simulink model "sedemo_shared_buffer_mgmt"  (Simulink 7.5)
settings: Solver=VariableStepDiscrete  StartTime=0.0  StopTime=10  MaxStep=inf  RelTol=1e-3
undefined symbols (not defined in the file or in its folder): des_subsystemblock, des_subsysteminport, des_subsystemoutport, des_subsystemsupportblock
libraries: simeventstranslate1 x25, simeventssink1 x23, simeventsrouting1 x9, simeventsgates1 x6, simeventsattributes2 x6, simeventsgenerators1 x6, simeventsserver1 x3, simeventsqueue1 x2, simulink x1, simeventsinfo x1
(part 1 of 4)
settings Model: Creator=The MathWorks Inc.  ExtModeAutoUpdateStatusClock=off
settings DataIOCC: SaveOutput=off  SignalLogging=off  SaveTime=off
settings OptimizationCC: InitFltsAndDblsToZero=on
settings DebuggingCC: AlgebraicLoopMsg=error  SolverPrmCheckMsg=none  StrictBusMsg=Warning
settings GRTTargetCC: TargetFcnLib=ansi_tfl_tmw_new.mat
settings SimEventsCC: propDiagAttribOutput=0  propDiagFcnCallOutput=1  propDiagStatOutput=0

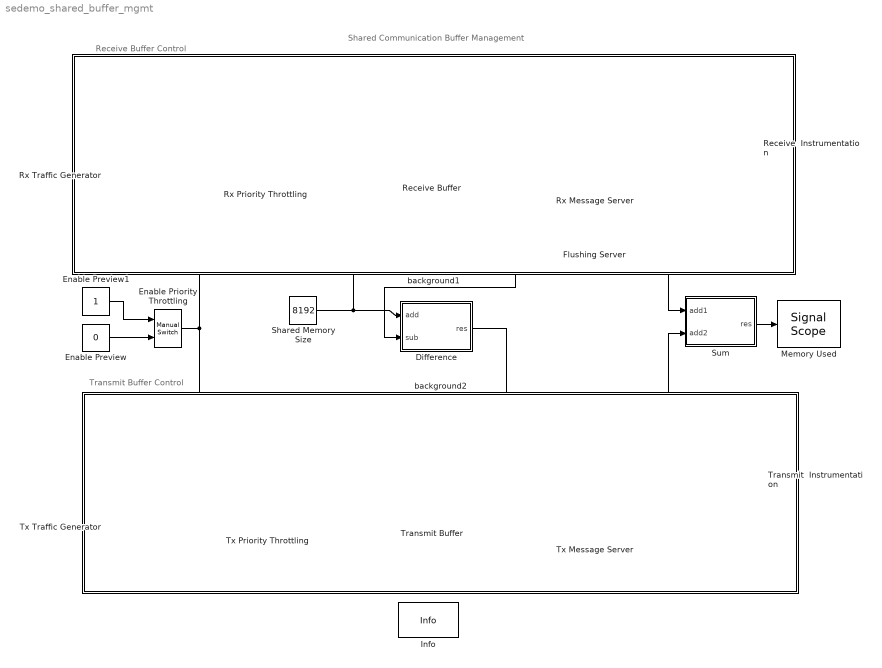
== system sedemo_shared_buffer_mgmt ==
  note: Shared Communication Buffer Management
  note: Receive Buffer Control
  note: Transmit Buffer Control
  Difference : Subsystem  LoadFcn=des_subsystemblock(gcb, 'load');  InitFcn=des_subsystemblock(gcb, 'init');  StartFcn=des_subsystemblock(gcb, 'start');  StopFcn=des_subsystemblock(gcb, 'stop');
      settings: CopyFcn=des_subsystemblock(gcb, 'copy');  DeleteFcn=des_subsystemblock(gcb, 'delete');  UndoDeleteFcn=des_subsystemblock(gcb, 'undodelete');  ModelCloseFcn=des_subsystemblock(gcb, 'modelclose');  PreSaveFcn=des_subsystemblock(gcb, 'presave');  NameChangeFcn=des_subsystemblock(gcb, 'namechange');  ParentCloseFcn=des_subsystemblock(gcb, 'parentclose');  ErrorFcn=des_subsystemerror
  Enable Preview : Constant  Value=0  OutDataType=sfix(16)  OutScaling=2^0
  Enable Preview1 : Constant  OutDataType=sfix(16)  OutScaling=2^0
  Enable Priority Throttling : simulink/Signal Routing/Manual Switch  SystemSampleTime=-1  sw=1  action=0  varsize=off
  Flushing Server : simeventsserver1/Single Server  Priority=1  SystemSampleTime=-1  ServiceTimeFrom=Dialog  ServiceTime=.01  AttributeName=ServiceTime  PriorityServiceCompletion=500  PermitPreemption=off  SortingAttributeName=PriorityAttributeName  SortingDirection=Ascending  WriteToAttribute=off  ResidualAttributeName=ResidualServiceTime  CreateAttribute=on  EnableTOPort=off  StatNumberDeparted=Off  StatNumberInBlock=Off  StatNumberPreempted=Off  StatPendingEntity=Off  StatAverageWait=Off  StatUtilization=Off  StatNumberTimedout=Off
  Info : simeventsinfo/Info  SystemSampleTime=-1
  Memory Used : simeventssink1/Signal Scope  Priority=1  SystemSampleTime=-1  PlotType=Stair  InputType=Signal  NumInputs=1  AttributeNameY=Count  XInputOptionSignal=Event time  XInputOptionEntity=Event time  AttributeNameX=Count  EnableEntityOutport=on  XMin=-0.1  XMax=10.1  XLimitExceededOption=Stretch axis limits  YLimitExceededOption=Stretch axis limits  AxisGrid=on  AxisLegend=off  LineDisables=""  LineColors="1  0  0"  LineStyles=-  LineMarkers=None  OpenScopeAtSimStart=on  Title=Total Memory Used  YLabel=Memory  XLabel=Time  FigurePosition=[598 478 273 129]  AxisZoom=off  DataStoreOption=Limited  DataPointsLimit=10000  StatNumberArrived=Off  ShowCountPlotted=off  ShowToolbar=off
      settings: YMin=-1.09  YMax=10
  Receive  Instrumentation : Subsystem
  Receive Buffer : Subsystem  mask(Variable Capacity, Variable Space per Entity Buffer){attribNameLength=space, thresholdLow=.35, thresholdHigh=.55}
      mask prompts: attribNameLength "Entity space from attribute:"; thresholdLow "Low threshold (fraction):"; thresholdHigh "High threshold (fraction):"
      mask help: Variable capacity queue that allows entities to occupy a variable amount of space per entitiy. The amount of space from an entity is specified from the attribute named in the dialog.
      mask init:
      | % Get attribute name to use for space needed for each entity
      | % and use it to set the attribute name for 'Get Attribute'
      | % and 'Get Attribute1' block
      | name = get_param(gcb,'attribNameLength');
      | set_param([gcb '/Get Attribute'],'AttributeName',name);
      | set_param([gcb '/Get Attribute1'],'AttributeName',name);
      mask Display:
      | color('blue')
      | text(35,67,'Variable Space\nper Entity and\nFlushing')
  Rx Message Server : simeventsserver1/Single Server  Priority=1  SystemSampleTime=-1  ServiceTimeFrom=Dialog  ServiceTime=.23  AttributeName=ServiceTime  PriorityServiceCompletion=500  PermitPreemption=off  SortingAttributeName=PriorityAttributeName  SortingDirection=Ascending  WriteToAttribute=off  ResidualAttributeName=ResidualServiceTime  CreateAttribute=on  EnableTOPort=off  StatNumberDeparted=On  StatNumberInBlock=Off  StatNumberPreempted=Off  StatPendingEntity=Off  StatAverageWait=Off  StatUtilization=Off  StatNumberTimedout=Off
  Rx Priority Throttling : Subsystem
  Rx Traffic Generator : Subsystem
  Shared Memory Size : Constant  Value=8192  OutDataType=sfix(16)  OutScaling=2^0
  Sum : Subsystem  LoadFcn=des_subsystemblock(gcb, 'load');  InitFcn=des_subsystemblock(gcb, 'init');  StartFcn=des_subsystemblock(gcb, 'start');  StopFcn=des_subsystemblock(gcb, 'stop');
      settings: CopyFcn=des_subsystemblock(gcb, 'copy');  DeleteFcn=des_subsystemblock(gcb, 'delete');  UndoDeleteFcn=des_subsystemblock(gcb, 'undodelete');  ModelCloseFcn=des_subsystemblock(gcb, 'modelclose');  PreSaveFcn=des_subsystemblock(gcb, 'presave');  NameChangeFcn=des_subsystemblock(gcb, 'namechange');  ParentCloseFcn=des_subsystemblock(gcb, 'parentclose');  ErrorFcn=des_subsystemerror
  Transmit  Instrumentation : Subsystem
  Transmit Buffer : Subsystem  mask(Variable Capacity, Variable Space per Entity Buffer){attribNameLength=space, thresholdLow=.4, thresholdHigh=.6}
      mask prompts: attribNameLength "Entity space from attribute:"; thresholdLow "Low threshold (fraction):"; thresholdHigh "High threshold (fraction):"
      mask help: Variable capacity queue that allows entities to occupy a variable amount of space per entitiy. The amount of space from an entity is specified from the attribute named in the dialog.
      mask init: same as sedemo_shared_buffer_mgmt/Receive Buffer
      mask Display:
      | color('blue')
      | text(35,67,'Variable Capacity\nwith Variable Space\nper Entity')
  Tx Message Server : simeventsserver1/Single Server  Priority=1  SystemSampleTime=-1  ServiceTimeFrom=Dialog  ServiceTime=.23  AttributeName=ServiceTime  PriorityServiceCompletion=500  PermitPreemption=off  SortingAttributeName=PriorityAttributeName  SortingDirection=Ascending  WriteToAttribute=off  ResidualAttributeName=ResidualServiceTime  CreateAttribute=on  EnableTOPort=off  StatNumberDeparted=On  StatNumberInBlock=Off  StatNumberPreempted=Off  StatPendingEntity=Off  StatAverageWait=Off  StatUtilization=Off  StatNumberTimedout=Off
  Tx Priority Throttling : Subsystem
  Tx Traffic Generator : Subsystem
  background1 : Subsystem
      mask Display: disp('')
  background2 : Subsystem
      mask Display: disp('')
  wires:
  Rx Message Server/1 -> Receive  Instrumentation/6(Num Served)
  Receive Buffer/1(#n) -> Receive  Instrumentation/1(Msgs)
  Receive Buffer/2(Mem) -> Receive  Instrumentation/2(Mem Used), Sum/1(add1), Difference/2(sub)
  Receive Buffer/3(high) -> Receive  Instrumentation/3(High), Rx Priority Throttling/3(drop high)
  Receive Buffer/4(#fl) -> Receive  Instrumentation/4(Num fl)
  Receive Buffer/5(low) -> Rx Priority Throttling/1(drop low), Receive  Instrumentation/5(low)
  Tx Message Server/1 -> Transmit  Instrumentation/6(Num Served)
  Transmit Buffer/1(#n) -> Transmit  Instrumentation/1(Msgs)
  Transmit Buffer/2(Mem) -> Sum/2(add2), Transmit  Instrumentation/2(Mem Used)
  Transmit Buffer/3(high) -> Tx Priority Throttling/3(drop high), Transmit  Instrumentation/3(high)
  Transmit Buffer/4(#fl) -> Transmit  Instrumentation/4(Num fl)
  Transmit Buffer/5(low) -> Tx Priority Throttling/1(drop low), Transmit  Instrumentation/5(low)
  Difference/1(res) -> Transmit Buffer/1(cap), Transmit  Instrumentation/7(Thresh)
  Sum/1(res) -> Memory Used/1
  Shared Memory Size/1 -> Difference/1(add), Receive Buffer/1(cap), Receive  Instrumentation/7(Thresh)
  Enable Preview1/1 -> Enable Priority Throttling/1
  Enable Preview/1 -> Enable Priority Throttling/2
  Enable Priority Throttling/1 -> Rx Priority Throttling/2(enable), Tx Priority Throttling/2(enable)
  connections:
  Receive Buffer/RConn1 -- Rx Message Server/LConn1
  Receive  Instrumentation/LConn1 -- Rx Message Server/RConn1
  Rx Traffic Generator/RConn1 -- Rx Priority Throttling/LConn1
  Rx Priority Throttling/RConn1 -- Receive Buffer/LConn1
  Transmit  Instrumentation/LConn1 -- Tx Message Server/RConn1
  Transmit Buffer/RConn1 -- Tx Message Server/LConn1
  Tx Traffic Generator/RConn1 -- Tx Priority Throttling/LConn1
  Tx Priority Throttling/RConn1 -- Transmit Buffer/LConn1
  Receive Buffer/RConn2 -- Flushing Server/LConn1
  Flushing Server/RConn1 -- Receive  Instrumentation/LConn2

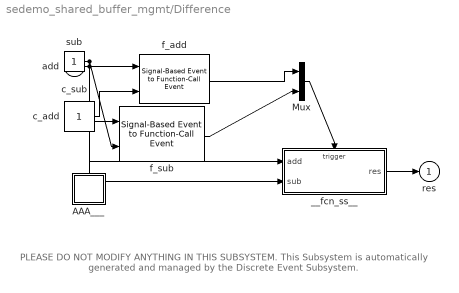
== system sedemo_shared_buffer_mgmt/Difference ==
  note: PLEASE DO NOT MODIFY ANYTHING IN THIS SUBSYSTEM.
      | This Subsystem is automatically generated and
      | managed by the Discrete Event Subsystem.
  add : Inport  DataType=double  OutDataType=sfix(16)  OutScaling=2^0  OutDataTypeStr=double
  sub : Inport  Port=2  DataType=double  OutDataType=sfix(16)  OutScaling=2^0  OutDataTypeStr=double
  AAA___ : Subsystem  LoadFcn=des_subsystemsupportblock(gcb, 'load');  InitFcn=des_subsystemsupportblock(gcb, 'init');  StartFcn=des_subsystemsupportblock(gcb, 'start');  StopFcn=des_subsystemsupportblock(gcb, 'stop');
      settings: CopyFcn=des_subsystemsupportblock(gcb, 'copy');  DeleteFcn=des_subsystemsupportblock(gcb, 'delete');  UndoDeleteFcn=des_subsystemsupportblock(gcb, 'undodelete');  ModelCloseFcn=des_subsystemsupportblock(gcb, 'modelclose');  PreSaveFcn=des_subsystemsupportblock(gcb, 'presave');  NameChangeFcn=des_subsystemsupportblock(gcb, 'namechange');  OpenFcn=des_subsystemsupportblock(gcb, 'open');  ParentCloseFcn=des_subsystemsupportblock(gcb, 'parentclose');
  Mux : Mux  Inputs=2
  __fcn_ss__ : Subsystem  TreatAsAtomicUnit=on
      settings: PropExecContextOutsideSubsystem=on
  c_add : Constant  OutDataType=sfix(16)  OutScaling=2^0
  c_sub : Constant  OutDataType=sfix(16)  OutScaling=2^0
  f_add : simeventstranslate1/Signal-Based Event to Function-Call Event  Priority=1  SystemSampleTime=-1  GenerateFunctionCallUpon=Sample time hit from port ts  SignalEdgeOption=Rising  EnableE1Port=on  EnableF2Port=off  EnableE2Port=off  SpecifyEventPriority=off  PriorityFunctionCall=20  FunctionCallDelayFrom=Dialog  DelayFunctionCall=0  StatNumberF1Calls=Off  StatNumberF2Calls=Off  MaskBlockType=DESS_EVENT_PORT
  f_sub : simeventstranslate1/Signal-Based Event to Function-Call Event  Priority=1  SystemSampleTime=-1  GenerateFunctionCallUpon=Sample time hit from port ts  SignalEdgeOption=Rising  EnableE1Port=on  EnableF2Port=off  EnableE2Port=off  SpecifyEventPriority=off  PriorityFunctionCall=20  FunctionCallDelayFrom=Dialog  DelayFunctionCall=0  StatNumberF1Calls=Off  StatNumberF2Calls=Off  MaskBlockType=DESS_EVENT_PORT
  res : Outport  OutDataType=sfix(16)  OutScaling=2^0
  wires:
  __fcn_ss__/1(res) -> res/1
  f_add/1 -> Mux/1
  c_add/1 -> f_add/2
  Mux/1 -> __fcn_ss__/Trigger
  f_sub/1 -> Mux/2
  c_sub/1 -> f_sub/2
  add/1 -> f_add/1, __fcn_ss__/1(add)
  sub/1 -> f_sub/1, __fcn_ss__/2(sub)

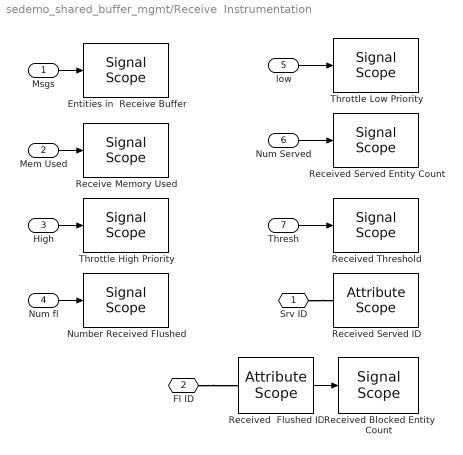
== system sedemo_shared_buffer_mgmt/Receive  Instrumentation ==
  Msgs : Inport  OutDataType=sfix(16)  OutScaling=2^0
  Mem Used : Inport  Port=2  OutDataType=sfix(16)  OutScaling=2^0
  High : Inport  Port=3  OutDataType=sfix(16)  OutScaling=2^0
  Num fl : Inport  Port=4  OutDataType=sfix(16)  OutScaling=2^0
  low : Inport  Port=5  OutDataType=sfix(16)  OutScaling=2^0
  Num Served : Inport  Port=6  OutDataType=sfix(16)  OutScaling=2^0
  Thresh : Inport  Port=7  OutDataType=sfix(16)  OutScaling=2^0
  Entities in  Receive Buffer : simeventssink1/Signal Scope  Priority=1  SystemSampleTime=-1  PlotType=Stair  InputType=Signal  NumInputs=1  AttributeNameY=Count  XInputOptionSignal=Event time  XInputOptionEntity=Event time  AttributeNameX=Count  EnableEntityOutport=on  XMin=0  XMax=10  XLimitExceededOption=Stretch axis limits  YLimitExceededOption=Stretch axis limits  AxisGrid=on  AxisLegend=off  LineDisables=""  LineColors=b  LineStyles=-  LineMarkers=.  OpenScopeAtSimStart=on  Title=Messages in Receive Buffer  YLabel=Num. Messages  XLabel=Time  FigurePosition=[28 477 268 129]  AxisZoom=off  DataStoreOption=Limited  DataPointsLimit=10000  StatNumberArrived=Off  ShowCountPlotted=off  ShowToolbar=off
      settings: YMin=0  YMax=10
  Number Received Flushed : simeventssink1/Signal Scope  Priority=1  SystemSampleTime=-1  PlotType=Stair  InputType=Signal  NumInputs=1  AttributeNameY=Count  XInputOptionSignal=Event time  XInputOptionEntity=Event time  AttributeNameX=Count  EnableEntityOutport=on  XMin=0  XMax=10  XLimitExceededOption=Stretch axis limits  YLimitExceededOption=Stretch axis limits  AxisGrid=on  AxisLegend=off  LineDisables=""  LineColors="1  0  0"  LineStyles=-  LineMarkers=None  OpenScopeAtSimStart=off  Title=Number Received Entities Flushed  YLabel=Number Flushed  XLabel=Time  FigurePosition=[883 418 268 129]  AxisZoom=off  DataStoreOption=Limited  DataPointsLimit=10000  StatNumberArrived=Off  ShowCountPlotted=off  ShowToolbar=on
      settings: YMin=0  YMax=10
  Receive Memory Used : simeventssink1/Signal Scope  Priority=1  SystemSampleTime=-1  PlotType=Stair  InputType=Signal  NumInputs=1  AttributeNameY=Count  XInputOptionSignal=Event time  XInputOptionEntity=Event time  AttributeNameX=Count  EnableEntityOutport=on  XMin=-0.1  XMax=10.1  XLimitExceededOption=Stretch axis limits  YLimitExceededOption=Stretch axis limits  AxisGrid=on  AxisLegend=off  LineDisables=""  LineColors="1  0  0"  LineStyles=-  LineMarkers=None  OpenScopeAtSimStart=on  Title=Receive Memory Used  YLabel=Memory  XLabel=Time  FigurePosition=[304 478 285 129]  AxisZoom=off  DataStoreOption=Limited  DataPointsLimit=10000  StatNumberArrived=Off  ShowCountPlotted=off  ShowToolbar=off
      settings: YMin=-1.09  YMax=10
  Received  Flushed ID : simeventssink1/Attribute Scope  Priority=1  SystemSampleTime=-1  PlotType=Stair  InputType=Attribute  NumInputs=1  AttributeNameY=count  XInputOptionSignal=Event time  XInputOptionEntity=Event time  AttributeNameX=Count  EnableEntityOutport=off  XMin=0  XMax=10  XLimitExceededOption=Stretch axis limits  YLimitExceededOption=Stretch axis limits  AxisGrid=on  AxisLegend=off  LineDisables=""  LineColors=b  LineStyles=-  LineMarkers=.  OpenScopeAtSimStart=off  Title=ID of Received Entities Flushed  YLabel=ID  XLabel=Time  FigurePosition=[783 206 237 129]  AxisZoom=off  DataStoreOption=Limited  DataPointsLimit=10000  StatNumberArrived=On  ShowCountPlotted=off  ShowToolbar=on
      settings: YMin=0  YMax=10
  Received Blocked Entity Count : simeventssink1/Signal Scope  Priority=1  SystemSampleTime=-1  PlotType=Stair  InputType=Signal  NumInputs=1  AttributeNameY=Count  XInputOptionSignal=Event time  XInputOptionEntity=Event time  AttributeNameX=Count  EnableEntityOutport=on  XMin=-0.1  XMax=10.1  XLimitExceededOption=Stretch axis limits  YLimitExceededOption=Stretch axis limits  AxisGrid=on  AxisLegend=off  LineDisables=""  LineColors=b  LineStyles=-  LineMarkers=.  OpenScopeAtSimStart=off  Title=Received Flushed Entity Count  YLabel=Entities Flushed  XLabel=Time  FigurePosition=[596 206 280 129]  AxisZoom=off  DataStoreOption=Limited  DataPointsLimit=10000  StatNumberArrived=Off  ShowCountPlotted=off  ShowToolbar=on
      settings: YMin=-0.19  YMax=19.19
  Received Served Entity Count : simeventssink1/Signal Scope  Priority=1  SystemSampleTime=-1  PlotType=Stair  InputType=Signal  NumInputs=1  AttributeNameY=Count  XInputOptionSignal=Event time  XInputOptionEntity=Event time  AttributeNameX=Count  EnableEntityOutport=on  XMin=0  XMax=10  XLimitExceededOption=Stretch axis limits  YLimitExceededOption=Stretch axis limits  AxisGrid=on  AxisLegend=off  LineDisables=""  LineColors=b  LineStyles=-  LineMarkers=.  OpenScopeAtSimStart=off  Title=Received Served Entity Count  YLabel=Entities Served  XLabel=Time  FigurePosition=[596 418 279 129]  AxisZoom=off  DataStoreOption=Limited  DataPointsLimit=10000  StatNumberArrived=Off  ShowCountPlotted=off  ShowToolbar=on
      settings: YMin=0  YMax=10
  Received Served ID : simeventssink1/Attribute Scope  Priority=1  SystemSampleTime=-1  PlotType=Stair  InputType=Attribute  NumInputs=1  AttributeNameY=count  XInputOptionSignal=Event time  XInputOptionEntity=Event time  AttributeNameX=Count  EnableEntityOutport=off  XMin=0  XMax=10  XLimitExceededOption=Stretch axis limits  YLimitExceededOption=Stretch axis limits  AxisGrid=on  AxisLegend=off  LineDisables=""  LineColors=b  LineStyles=-  LineMarkers=.  OpenScopeAtSimStart=off  Title=ID of Receive Entities Served  YLabel=ID  XLabel=Time  FigurePosition=[884 206 243 129]  AxisZoom=off  DataStoreOption=Limited  DataPointsLimit=10000  StatNumberArrived=Off  ShowCountPlotted=off  ShowToolbar=on
      settings: YMin=0  YMax=10
  Received Threshold : simeventssink1/Signal Scope  Priority=1  SystemSampleTime=-1  PlotType=Stair  InputType=Signal  NumInputs=1  AttributeNameY=Count  XInputOptionSignal=Event time  XInputOptionEntity=Event time  AttributeNameX=Count  EnableEntityOutport=on  XMin=0  XMax=10  XLimitExceededOption=Stretch axis limits  YLimitExceededOption=Stretch axis limits  AxisGrid=on  AxisLegend=off  LineDisables=""  LineColors="1  0  0"  LineStyles=-  LineMarkers=None  OpenScopeAtSimStart=off  Title=Threshold for Transmit Memory Used  YLabel=Threshold  XLabel=Time  FigurePosition=[27 206 272 129]  AxisZoom=off  DataStoreOption=Limited  DataPointsLimit=10000  StatNumberArrived=Off  ShowCountPlotted=off  ShowToolbar=on
      settings: YMin=0  YMax=10
  Throttle High Priority : simeventssink1/Signal Scope  Priority=1  SystemSampleTime=-1  PlotType=Stair  InputType=Signal  NumInputs=1  AttributeNameY=Count  XInputOptionSignal=Event time  XInputOptionEntity=Event time  AttributeNameX=Count  EnableEntityOutport=on  XMin=0  XMax=10  XLimitExceededOption=Stretch axis limits  YLimitExceededOption=Stretch axis limits  AxisGrid=on  AxisLegend=off  LineDisables=""  LineColors="1  0  0"  LineStyles=-  LineMarkers=None  OpenScopeAtSimStart=off  Title=Throttle High Priority Messages  YLabel=Enable Flush  XLabel=Time  FigurePosition=[303 418 283 129]  AxisZoom=off  DataStoreOption=Limited  DataPointsLimit=10000  StatNumberArrived=Off  ShowCountPlotted=off  ShowToolbar=on
      settings: YMin=0  YMax=10
  Throttle Low Priority : simeventssink1/Signal Scope  Priority=1  SystemSampleTime=-1  PlotType=Stair  InputType=Signal  NumInputs=1  AttributeNameY=Count  XInputOptionSignal=Event time  XInputOptionEntity=Event time  AttributeNameX=Count  EnableEntityOutport=on  XMin=0  XMax=10  XLimitExceededOption=Stretch axis limits  YLimitExceededOption=Stretch axis limits  AxisGrid=on  AxisLegend=off  LineDisables=""  LineColors="1  0  0"  LineStyles=-  LineMarkers=None  OpenScopeAtSimStart=off  Title=Throttle Low Priority Message  YLabel=Status  XLabel=Time  FigurePosition=[307 418 268 129]  AxisZoom=off  DataStoreOption=Limited  DataPointsLimit=10000  StatNumberArrived=Off  ShowCountPlotted=off  ShowToolbar=on
      settings: YMin=0  YMax=10
  Srv ID : PMIOPort  Port=1  Side=Left
  Fl ID : PMIOPort  Port=2  Side=Left
  wires:
  Received  Flushed ID/1 -> Received Blocked Entity Count/1
  low/1 -> Throttle Low Priority/1
  Thresh/1 -> Received Threshold/1
  Mem Used/1 -> Receive Memory Used/1
  Msgs/1 -> Entities in  Receive Buffer/1
  High/1 -> Throttle High Priority/1
  Num fl/1 -> Number Received Flushed/1
  Num Served/1 -> Received Served Entity Count/1
  connections:
  Srv ID/RConn1 -- Received Served ID/LConn1
  Fl ID/RConn1 -- Received  Flushed ID/LConn1

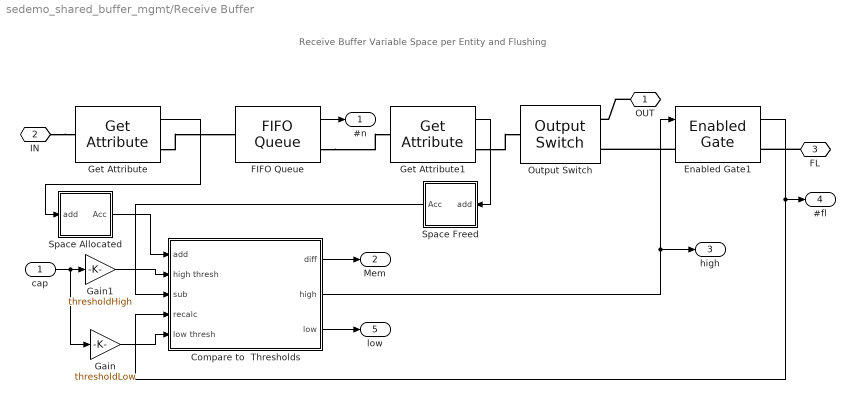
== system sedemo_shared_buffer_mgmt/Receive Buffer ==
  note: Receive Buffer
      | Variable Space per Entity and Flushing
  cap : Inport  OutDataType=sfix(16)  OutScaling=2^0
  Compare to  Thresholds : Subsystem  LoadFcn=des_subsystemblock(gcb, 'load');  InitFcn=des_subsystemblock(gcb, 'init');  StartFcn=des_subsystemblock(gcb, 'start');  StopFcn=des_subsystemblock(gcb, 'stop');
      settings: CopyFcn=des_subsystemblock(gcb, 'copy');  DeleteFcn=des_subsystemblock(gcb, 'delete');  UndoDeleteFcn=des_subsystemblock(gcb, 'undodelete');  ModelCloseFcn=des_subsystemblock(gcb, 'modelclose');  PreSaveFcn=des_subsystemblock(gcb, 'presave');  NameChangeFcn=des_subsystemblock(gcb, 'namechange');  ParentCloseFcn=des_subsystemblock(gcb, 'parentclose');  ErrorFcn=des_subsystemerror
  Enabled Gate1 : simeventsgates1/Enabled Gate  Priority=1  SystemSampleTime=-1  SpecifyEventPriority=off  PriorityGateEnableOpenClose=500  StatNumberDeparted=On
  FIFO Queue : simeventsqueue1/FIFO Queue  Priority=1  SystemSampleTime=-1  Capacity=inf  EnableTOPort=off  StatNumberDeparted=Off  StatNumberInBlock=On  StatPendingEntity=Off  StatAverageWait=Off  StatAverageQueueLength=Off  StatNumberTimedout=Off
  Gain : Gain  Gain=thresholdLow  ParameterDataType=sfix(16)  ParameterScaling=2^0  OutDataType=sfix(16)  OutScaling=2^0
  Gain1 : Gain  Gain=thresholdHigh  ParameterDataType=sfix(16)  ParameterScaling=2^0  OutDataType=sfix(16)  OutScaling=2^0
  Get Attribute : simeventsattributes2/Get Attribute  Priority=1  DialogController=des_ddg_create  DialogControllerArgs=DataTag41  SystemSampleTime=-1  AttributeName=space  AttributeMissing=Error  AttributeDefaultValue=1  AttributeSendTiming=After entity departure  AttributeTreatAsVector=1  StatNumberDeparted=Off  EvaluatedDefaultAttributeValue={[]}
  Get Attribute1 : simeventsattributes2/Get Attribute  Priority=1  DialogController=des_ddg_create  DialogControllerArgs=DataTag43  SystemSampleTime=-1  AttributeName=space  AttributeMissing=Error  AttributeDefaultValue=1  AttributeSendTiming=After entity departure  AttributeTreatAsVector=1  StatNumberDeparted=Off  EvaluatedDefaultAttributeValue={[]}
  Output Switch : simeventsrouting1/Output Switch  Priority=1  SystemSampleTime=-1  NumberOutputPorts=2  SwitchingCriterion=First port that is not blocked  InitialSeed=34567  AttributeName=Attribute1  InitialConditionsOpt=on  InitialConditions=1  EntityBufferOpt=on  SpecifyEventPriority=off  PriorityOutputSwitchSelectPort=4100  TimeoutPortOpt=off  StatNumberDeparted=Off  StatNumberTimedOut=Off  StatPendingEntity=Off  StatLastDeparturePort=Off  EvaluatedNumPorts=2
  Space Allocated : Subsystem  LoadFcn=des_subsystemblock(gcb, 'load');  InitFcn=des_subsystemblock(gcb, 'init');  StartFcn=des_subsystemblock(gcb, 'start');  StopFcn=des_subsystemblock(gcb, 'stop');
      settings: CopyFcn=des_subsystemblock(gcb, 'copy');  DeleteFcn=des_subsystemblock(gcb, 'delete');  UndoDeleteFcn=des_subsystemblock(gcb, 'undodelete');  ModelCloseFcn=des_subsystemblock(gcb, 'modelclose');  PreSaveFcn=des_subsystemblock(gcb, 'presave');  NameChangeFcn=des_subsystemblock(gcb, 'namechange');  ParentCloseFcn=des_subsystemblock(gcb, 'parentclose');  ErrorFcn=des_subsystemerror
  Space Freed : Subsystem  LoadFcn=des_subsystemblock(gcb, 'load');  InitFcn=des_subsystemblock(gcb, 'init');  StartFcn=des_subsystemblock(gcb, 'start');  StopFcn=des_subsystemblock(gcb, 'stop');
      settings: CopyFcn=des_subsystemblock(gcb, 'copy');  DeleteFcn=des_subsystemblock(gcb, 'delete');  UndoDeleteFcn=des_subsystemblock(gcb, 'undodelete');  ModelCloseFcn=des_subsystemblock(gcb, 'modelclose');  PreSaveFcn=des_subsystemblock(gcb, 'presave');  NameChangeFcn=des_subsystemblock(gcb, 'namechange');  ParentCloseFcn=des_subsystemblock(gcb, 'parentclose');  ErrorFcn=des_subsystemerror
  OUT : PMIOPort  Port=1  Side=Right
  IN : PMIOPort  Port=2  Side=Left
  FL : PMIOPort  Port=3  Side=Right
  #n : Outport  OutDataType=sfix(16)  OutScaling=2^0
  Mem : Outport  Port=2  OutDataType=sfix(16)  OutScaling=2^0
  high : Outport  Port=3  OutDataType=sfix(16)  OutScaling=2^0
  #fl : Outport  Port=4  OutDataType=sfix(16)  OutScaling=2^0
  low : Outport  Port=5  OutDataType=sfix(16)  OutScaling=2^0
  wires:
  Get Attribute1/1 -> Space Freed/1(add)
  Get Attribute/1 -> Space Allocated/1(add)
  Space Freed/1(Acc) -> Compare to  Thresholds/3(sub)
  Space Allocated/1(Acc) -> Compare to  Thresholds/1(add)
  Compare to  Thresholds/2(high) -> Enabled Gate1/1, high/1
  Enabled Gate1/1 -> Compare to  Thresholds/4(recalc), #fl/1
  FIFO Queue/1 -> #n/1
  Compare to  Thresholds/1(diff) -> Mem/1
  Gain/1 -> Compare to  Thresholds/5(low thresh)
  Compare to  Thresholds/3(low) -> low/1
  cap/1 -> Gain/1, Gain1/1
  Gain1/1 -> Compare to  Thresholds/2(high thresh)
  connections:
  Enabled Gate1/LConn1 -- Output Switch/RConn2
  Get Attribute/RConn1 -- FIFO Queue/LConn1
  FIFO Queue/RConn1 -- Get Attribute1/LConn1
  OUT/RConn1 -- Output Switch/RConn1
  IN/RConn1 -- Get Attribute/LConn1
  FL/RConn1 -- Enabled Gate1/RConn1
  Get Attribute1/RConn1 -- Output Switch/LConn1

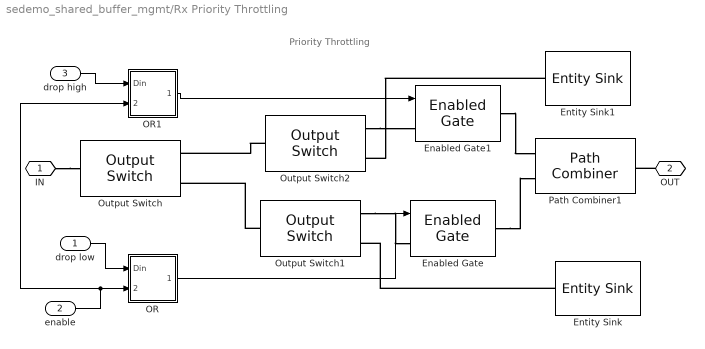
== system sedemo_shared_buffer_mgmt/Rx Priority Throttling ==
  note: Priority Throttling
  drop low : Inport  OutDataType=sfix(16)  OutScaling=2^0
  enable : Inport  Port=2  OutDataType=sfix(16)  OutScaling=2^0
  drop high : Inport  Port=3  OutDataType=sfix(16)  OutScaling=2^0
  Enabled Gate : simeventsgates1/Enabled Gate  Priority=1  SystemSampleTime=-1  SpecifyEventPriority=off  PriorityGateEnableOpenClose=2000  StatNumberDeparted=Off
  Enabled Gate1 : simeventsgates1/Enabled Gate  Priority=1  SystemSampleTime=-1  SpecifyEventPriority=off  PriorityGateEnableOpenClose=2000  StatNumberDeparted=Off
  Entity Sink : simeventssink1/Entity Sink  Priority=1  SystemSampleTime=-1  AvailableForArrivals=on  StatNumberArrived=Off
  Entity Sink1 : simeventssink1/Entity Sink  Priority=1  SystemSampleTime=-1  AvailableForArrivals=on  StatNumberArrived=Off
  OR : Subsystem  LoadFcn=des_subsystemblock(gcb, 'load');  InitFcn=des_subsystemblock(gcb, 'init');  StartFcn=des_subsystemblock(gcb, 'start');  StopFcn=des_subsystemblock(gcb, 'stop');
      settings: CopyFcn=des_subsystemblock(gcb, 'copy');  DeleteFcn=des_subsystemblock(gcb, 'delete');  UndoDeleteFcn=des_subsystemblock(gcb, 'undodelete');  ModelCloseFcn=des_subsystemblock(gcb, 'modelclose');  PreSaveFcn=des_subsystemblock(gcb, 'presave');  NameChangeFcn=des_subsystemblock(gcb, 'namechange');  ParentCloseFcn=des_subsystemblock(gcb, 'parentclose');  ErrorFcn=des_subsystemerror
  OR1 : Subsystem  LoadFcn=des_subsystemblock(gcb, 'load');  InitFcn=des_subsystemblock(gcb, 'init');  StartFcn=des_subsystemblock(gcb, 'start');  StopFcn=des_subsystemblock(gcb, 'stop');
      settings: CopyFcn=des_subsystemblock(gcb, 'copy');  DeleteFcn=des_subsystemblock(gcb, 'delete');  UndoDeleteFcn=des_subsystemblock(gcb, 'undodelete');  ModelCloseFcn=des_subsystemblock(gcb, 'modelclose');  PreSaveFcn=des_subsystemblock(gcb, 'presave');  NameChangeFcn=des_subsystemblock(gcb, 'namechange');  ParentCloseFcn=des_subsystemblock(gcb, 'parentclose');  ErrorFcn=des_subsystemerror
  Output Switch : simeventsrouting1/Output Switch  Priority=1  SystemSampleTime=-1  NumberOutputPorts=2  SwitchingCriterion=From attribute  InitialSeed=34567  AttributeName=priority  InitialConditionsOpt=off  InitialConditions=1  EntityBufferOpt=off  SpecifyEventPriority=off  PriorityOutputSwitchSelectPort=4100  TimeoutPortOpt=off  StatNumberDeparted=Off  StatNumberTimedOut=Off  StatPendingEntity=Off  StatLastDeparturePort=Off  EvaluatedNumPorts=2
  Output Switch1 : simeventsrouting1/Output Switch  Priority=1  SystemSampleTime=-1  NumberOutputPorts=2  SwitchingCriterion=First port that is not blocked  InitialSeed=34567  AttributeName=priority  InitialConditionsOpt=off  InitialConditions=1  EntityBufferOpt=off  SpecifyEventPriority=off  PriorityOutputSwitchSelectPort=4100  TimeoutPortOpt=off  StatNumberDeparted=Off  StatNumberTimedOut=Off  StatPendingEntity=Off  StatLastDeparturePort=Off  EvaluatedNumPorts=2
  Output Switch2 : simeventsrouting1/Output Switch  Priority=1  SystemSampleTime=-1  NumberOutputPorts=2  SwitchingCriterion=First port that is not blocked  InitialSeed=34567  AttributeName=priority  InitialConditionsOpt=off  InitialConditions=1  EntityBufferOpt=off  SpecifyEventPriority=off  PriorityOutputSwitchSelectPort=4100  TimeoutPortOpt=off  StatNumberDeparted=Off  StatNumberTimedOut=Off  StatPendingEntity=Off  StatLastDeparturePort=Off  EvaluatedNumPorts=2
  Path Combiner1 : simeventsrouting1/Path Combiner  Priority=1  SystemSampleTime=-1  NumberInputPorts=2  InputPortPrecedence=IN1 port  InitialSeed=45675  SpecifyEventPriority=off  PriorityPathCombinerPortPrecedenceSelection=4100  StatNumberDeparted=Off  StatLastArrivalPort=Off  EvaluatedNumPorts=2
  IN : PMIOPort  Port=1  Side=Left
  OUT : PMIOPort  Port=2  Side=Right
  wires:
  drop low/1 -> OR/1(Din)
  enable/1 -> OR/2(Din1), OR1/2(Din1)
  OR/1(Dout) -> Enabled Gate/1
  drop high/1 -> OR1/1(Din)
  OR1/1(Dout) -> Enabled Gate1/1
  connections:
  IN/RConn1 -- Output Switch/LConn1
  OUT/RConn1 -- Path Combiner1/RConn1
  Enabled Gate/RConn1 -- Path Combiner1/LConn2
  Output Switch2/LConn1 -- Output Switch/RConn1
  Output Switch1/LConn1 -- Output Switch/RConn2
  Output Switch1/RConn1 -- Enabled Gate/LConn1
  Entity Sink/LConn1 -- Output Switch1/RConn2
  Output Switch2/RConn1 -- Enabled Gate1/LConn1
  Enabled Gate1/RConn1 -- Path Combiner1/LConn1
  Entity Sink1/LConn1 -- Output Switch2/RConn2

== system sedemo_shared_buffer_mgmt/Rx Traffic Generator ==
  Random Length : simeventsgenerators1/Signal Generators/Event-Based Random Number  SystemSampleTime=-1  distribution=Uniform  meanExp=1  minUnif=64  maxUnif=1518  pOneBern=0.25  pSuccessBino=0.5  numTrialBino=1  meanNorm=0  stdNorm=1  minTri=1  maxTri=3  modeTri=2  thresholdLogn=0  scaleLogn=1  shapeLogn=1  pSuccessGeo=0.5  meanPoiss=1  thresholdLogl=0  scaleLogl=1  thresholdGam=0  scaleGam=1  shapeGam=1  minBeta=0  maxBeta=1  shape1Beta=1  shape2Beta=1  minUnid=0  maxUnid=1  numValueUnid=2  thresholdWbl=0  scaleWbl=1  shapeWbl=1  valueVecCont=[0 1]  cdfVecCont=[0 1]  valueVecDisc=[1 2]  probVecDisc=priorityDist  seed=9538  IsProcessed=on  isConnected=1
  Random Priority : simeventsgenerators1/Signal Generators/Event-Based Random Number  SystemSampleTime=-1  distribution=Arbitrary discrete  meanExp=1  minUnif=1  maxUnif=1  pOneBern=0.25  pSuccessBino=0.5  numTrialBino=1  meanNorm=0  stdNorm=1  minTri=1  maxTri=3  modeTri=2  thresholdLogn=0  scaleLogn=1  shapeLogn=1  pSuccessGeo=0.5  meanPoiss=1  thresholdLogl=0  scaleLogl=1  thresholdGam=0  scaleGam=1  shapeGam=1  minBeta=0  maxBeta=1  shape1Beta=1  shape2Beta=1  minUnid=0  maxUnid=1  numValueUnid=2  thresholdWbl=0  scaleWbl=1  shapeWbl=1  valueVecCont=[0 1]  cdfVecCont=[0 1]  valueVecDisc=[1 2]  probVecDisc=[.3 .7]  seed=4925  IsProcessed=on  isConnected=1
  Set Attribute : simeventsattributes2/Set Attribute  Priority=1  DialogController=des_ddg_create  DialogControllerArgs=DataTag87  SystemSampleTime=-1  AttributeFrom=Signal port|Signal port|Signal port  AttributeName=space|priority|count  AttributeTreatAsVector=1|1|1  AttributeValue=1|1|1  AttributeCreate=on  StatNumberDeparted=Off  EvaluatedAttributeValue={[];[];[]}
  Time-Based Entity Generator : simeventsgenerators1/Entity Generators/Time-Based Entity Generator  Priority=1  DialogController=des_ddg_create  DialogControllerArgs=DataTag89  SystemSampleTime=-1  GenerateEntitiesUpon=Intergeneration time from dialog  Distribution=Exponential  Minimum=0  Maximum=.7  Mean=.1  InitialSeed=12345  Period=100  PriorityEntityGeneration=300  GenerateEntityAtSimulationStart=off  ResponseWhenBlocked=Pause generation  ResponseWhenUnblocked=Immediate restart  EntityType=Blank  StatNumberDeparted=On  StatPendingEntity=Off  StatAverageIntergenerationTime=Off
  OUT : PMIOPort  Port=1  Side=Right
  wires:
  Random Length/1 -> Set Attribute/1
  Time-Based Entity Generator/1 -> Set Attribute/3
  Random Priority/1 -> Set Attribute/2
  connections:
  Time-Based Entity Generator/RConn1 -- Set Attribute/LConn1
  OUT/RConn1 -- Set Attribute/RConn1

== system sedemo_shared_buffer_mgmt/Sum ==
  note: PLEASE DO NOT MODIFY ANYTHING IN THIS SUBSYSTEM.
      | This Subsystem is automatically generated and
      | managed by the Discrete Event Subsystem.
  add1 : Inport  DataType=double  OutDataType=sfix(16)  OutScaling=2^0  OutDataTypeStr=double
  add2 : Inport  Port=2  DataType=double  OutDataType=sfix(16)  OutScaling=2^0  OutDataTypeStr=double
  AAA___ : Subsystem  LoadFcn=des_subsystemsupportblock(gcb, 'load');  InitFcn=des_subsystemsupportblock(gcb, 'init');  StartFcn=des_subsystemsupportblock(gcb, 'start');  StopFcn=des_subsystemsupportblock(gcb, 'stop');
      settings: CopyFcn=des_subsystemsupportblock(gcb, 'copy');  DeleteFcn=des_subsystemsupportblock(gcb, 'delete');  UndoDeleteFcn=des_subsystemsupportblock(gcb, 'undodelete');  ModelCloseFcn=des_subsystemsupportblock(gcb, 'modelclose');  PreSaveFcn=des_subsystemsupportblock(gcb, 'presave');  NameChangeFcn=des_subsystemsupportblock(gcb, 'namechange');  OpenFcn=des_subsystemsupportblock(gcb, 'open');  ParentCloseFcn=des_subsystemsupportblock(gcb, 'parentclose');
  Mux : Mux  Inputs=2
  __fcn_ss__ : Subsystem  TreatAsAtomicUnit=on
      settings: PropExecContextOutsideSubsystem=on
  c_add1 : Constant  OutDataType=sfix(16)  OutScaling=2^0
  c_add2 : Constant  OutDataType=sfix(16)  OutScaling=2^0
  f_add1 : simeventstranslate1/Signal-Based Event to Function-Call Event  Priority=1  SystemSampleTime=-1  GenerateFunctionCallUpon=Sample time hit from port ts  SignalEdgeOption=Rising  EnableE1Port=on  EnableF2Port=off  EnableE2Port=off  SpecifyEventPriority=off  PriorityFunctionCall=20  FunctionCallDelayFrom=Dialog  DelayFunctionCall=0  StatNumberF1Calls=Off  StatNumberF2Calls=Off  MaskBlockType=DESS_EVENT_PORT
  f_add2 : simeventstranslate1/Signal-Based Event to Function-Call Event  Priority=1  SystemSampleTime=-1  GenerateFunctionCallUpon=Sample time hit from port ts  SignalEdgeOption=Rising  EnableE1Port=on  EnableF2Port=off  EnableE2Port=off  SpecifyEventPriority=off  PriorityFunctionCall=20  FunctionCallDelayFrom=Dialog  DelayFunctionCall=0  StatNumberF1Calls=Off  StatNumberF2Calls=Off  MaskBlockType=DESS_EVENT_PORT
  res : Outport  OutDataType=sfix(16)  OutScaling=2^0
  wires:
  __fcn_ss__/1(res) -> res/1
  f_add1/1 -> Mux/1
  c_add1/1 -> f_add1/2
  Mux/1 -> __fcn_ss__/Trigger
  f_add2/1 -> Mux/2
  c_add2/1 -> f_add2/2
  add1/1 -> f_add1/1, __fcn_ss__/1(add1)
  add2/1 -> f_add2/1, __fcn_ss__/2(add2)

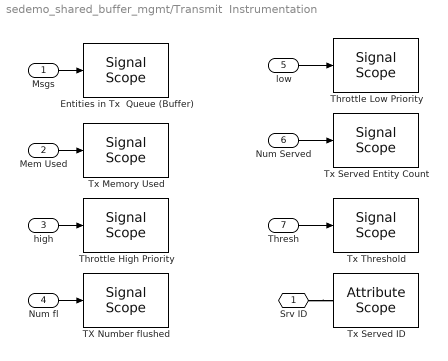
== system sedemo_shared_buffer_mgmt/Transmit  Instrumentation ==
  Msgs : Inport  OutDataType=sfix(16)  OutScaling=2^0
  Mem Used : Inport  Port=2  OutDataType=sfix(16)  OutScaling=2^0
  high : Inport  Port=3  OutDataType=sfix(16)  OutScaling=2^0
  Num fl : Inport  Port=4  OutDataType=sfix(16)  OutScaling=2^0
  low : Inport  Port=5  OutDataType=sfix(16)  OutScaling=2^0
  Num Served : Inport  Port=6  OutDataType=sfix(16)  OutScaling=2^0
  Thresh : Inport  Port=7  OutDataType=sfix(16)  OutScaling=2^0
  Entities in Tx  Queue (Buffer) : simeventssink1/Signal Scope  Priority=1  SystemSampleTime=-1  PlotType=Stair  InputType=Signal  NumInputs=1  AttributeNameY=Count  XInputOptionSignal=Event time  XInputOptionEntity=Event time  AttributeNameX=Count  EnableEntityOutport=on  XMin=0  XMax=10  XLimitExceededOption=Stretch axis limits  YLimitExceededOption=Stretch axis limits  AxisGrid=on  AxisLegend=off  LineDisables=""  LineColors=b  LineStyles=-  LineMarkers=.  OpenScopeAtSimStart=on  Title=Messages in Transmit Buffer  YLabel=Num. Message  XLabel=Time  FigurePosition=[27 290 268 129]  AxisZoom=off  DataStoreOption=Limited  DataPointsLimit=10000  StatNumberArrived=Off  ShowCountPlotted=off  ShowToolbar=off
      settings: YMin=0  YMax=10
  TX Number flushed : simeventssink1/Signal Scope  Priority=1  SystemSampleTime=-1  PlotType=Stair  InputType=Signal  NumInputs=1  AttributeNameY=Count  XInputOptionSignal=Event time  XInputOptionEntity=Event time  AttributeNameX=Count  EnableEntityOutport=on  XMin=0  XMax=10  XLimitExceededOption=Stretch axis limits  YLimitExceededOption=Stretch axis limits  AxisGrid=on  AxisLegend=off  LineDisables=""  LineColors="1  0  0"  LineStyles=-  LineMarkers=None  OpenScopeAtSimStart=off  Title=Number Transmit Entities Flushed  YLabel=Number Flushed  XLabel=Time  FigurePosition=[883 418 268 129]  AxisZoom=off  DataStoreOption=Limited  DataPointsLimit=10000  StatNumberArrived=Off  ShowCountPlotted=off  ShowToolbar=on
      settings: YMin=0  YMax=10
  Throttle High Priority : simeventssink1/Signal Scope  Priority=1  SystemSampleTime=-1  PlotType=Stair  InputType=Signal  NumInputs=1  AttributeNameY=Count  XInputOptionSignal=Event time  XInputOptionEntity=Event time  AttributeNameX=Count  EnableEntityOutport=on  XMin=0  XMax=10  XLimitExceededOption=Stretch axis limits  YLimitExceededOption=Stretch axis limits  AxisGrid=on  AxisLegend=off  LineDisables=""  LineColors="1  0  0"  LineStyles=-  LineMarkers=None  OpenScopeAtSimStart=off  Title=Throttle High Priority Message  YLabel=Enable Flush  XLabel=Time  FigurePosition=[303 418 283 129]  AxisZoom=off  DataStoreOption=Limited  DataPointsLimit=10000  StatNumberArrived=Off  ShowCountPlotted=off  ShowToolbar=on
      settings: YMin=0  YMax=10
  Throttle Low Priority : simeventssink1/Signal Scope  Priority=1  SystemSampleTime=-1  PlotType=Stair  InputType=Signal  NumInputs=1  AttributeNameY=Count  XInputOptionSignal=Event time  XInputOptionEntity=Event time  AttributeNameX=Count  EnableEntityOutport=on  XMin=0  XMax=10  XLimitExceededOption=Stretch axis limits  YLimitExceededOption=Stretch axis limits  AxisGrid=on  AxisLegend=off  LineDisables=""  LineColors="1  0  0"  LineStyles=-  LineMarkers=None  OpenScopeAtSimStart=off  Title=Throttle Low Priority Message  YLabel=Status  XLabel=Time  FigurePosition=[307 418 268 129]  AxisZoom=off  DataStoreOption=Limited  DataPointsLimit=10000  StatNumberArrived=Off  ShowCountPlotted=off  ShowToolbar=on
      settings: YMin=0  YMax=10
  Tx Memory Used : simeventssink1/Signal Scope  Priority=1  SystemSampleTime=-1  PlotType=Stair  InputType=Signal  NumInputs=1  AttributeNameY=Count  XInputOptionSignal=Event time  XInputOptionEntity=Event time  AttributeNameX=Count  EnableEntityOutport=on  XMin=-0.1  XMax=10.1  XLimitExceededOption=Stretch axis limits  YLimitExceededOption=Stretch axis limits  AxisGrid=on  AxisLegend=off  LineDisables=""  LineColors="1  0  0"  LineStyles=-  LineMarkers=None  OpenScopeAtSimStart=on  Title=Transmit Memory Used  YLabel=Memory  XLabel=Time  FigurePosition=[304 290 285 129]  AxisZoom=off  DataStoreOption=Limited  DataPointsLimit=10000  StatNumberArrived=Off  ShowCountPlotted=off  ShowToolbar=off
      settings: YMin=-1.09  YMax=10
  Tx Served Entity Count : simeventssink1/Signal Scope  Priority=1  SystemSampleTime=-1  PlotType=Stair  InputType=Signal  NumInputs=1  AttributeNameY=Count  XInputOptionSignal=Event time  XInputOptionEntity=Event time  AttributeNameX=Count  EnableEntityOutport=on  XMin=0  XMax=10  XLimitExceededOption=Stretch axis limits  YLimitExceededOption=Stretch axis limits  AxisGrid=on  AxisLegend=off  LineDisables=""  LineColors=b  LineStyles=-  LineMarkers=.  OpenScopeAtSimStart=off  Title=Transmit Served Entity Count  YLabel=Entities Served  XLabel=Time  FigurePosition=[596 418 279 129]  AxisZoom=off  DataStoreOption=Limited  DataPointsLimit=10000  StatNumberArrived=Off  ShowCountPlotted=off  ShowToolbar=on
      settings: YMin=0  YMax=10
  Tx Served ID : simeventssink1/Attribute Scope  Priority=1  SystemSampleTime=-1  PlotType=Stair  InputType=Attribute  NumInputs=1  AttributeNameY=count  XInputOptionSignal=Event time  XInputOptionEntity=Event time  AttributeNameX=Count  EnableEntityOutport=off  XMin=0  XMax=10  XLimitExceededOption=Stretch axis limits  YLimitExceededOption=Stretch axis limits  AxisGrid=on  AxisLegend=off  LineDisables=""  LineColors=b  LineStyles=-  LineMarkers=.  OpenScopeAtSimStart=off  Title=ID of Transmit Served Entities  YLabel=ID  XLabel=Time  FigurePosition=[884 206 243 129]  AxisZoom=off  DataStoreOption=Limited  DataPointsLimit=10000  StatNumberArrived=Off  ShowCountPlotted=off  ShowToolbar=on
      settings: YMin=0  YMax=10
  Tx Threshold : simeventssink1/Signal Scope  Priority=1  SystemSampleTime=-1  PlotType=Stair  InputType=Signal  NumInputs=1  AttributeNameY=Count  XInputOptionSignal=Event time  XInputOptionEntity=Event time  AttributeNameX=Count  EnableEntityOutport=on  XMin=0  XMax=10  XLimitExceededOption=Stretch axis limits  YLimitExceededOption=Stretch axis limits  AxisGrid=on  AxisLegend=off  LineDisables=""  LineColors="1  0  0"  LineStyles=-  LineMarkers=None  OpenScopeAtSimStart=on  Title=Threshold for Transmit Memory Used  YLabel=Threshold  XLabel=Time  FigurePosition=[598 291 272 129]  AxisZoom=off  DataStoreOption=Limited  DataPointsLimit=10000  StatNumberArrived=Off  ShowCountPlotted=off  ShowToolbar=off
      settings: YMin=0  YMax=10
  Srv ID : PMIOPort  Port=1  Side=Left
  wires:
  low/1 -> Throttle Low Priority/1
  Thresh/1 -> Tx Threshold/1
  Mem Used/1 -> Tx Memory Used/1
  Msgs/1 -> Entities in Tx  Queue (Buffer)/1
  high/1 -> Throttle High Priority/1
  Num fl/1 -> TX Number flushed/1
  Num Served/1 -> Tx Served Entity Count/1
  connections:
  Srv ID/RConn1 -- Tx Served ID/LConn1

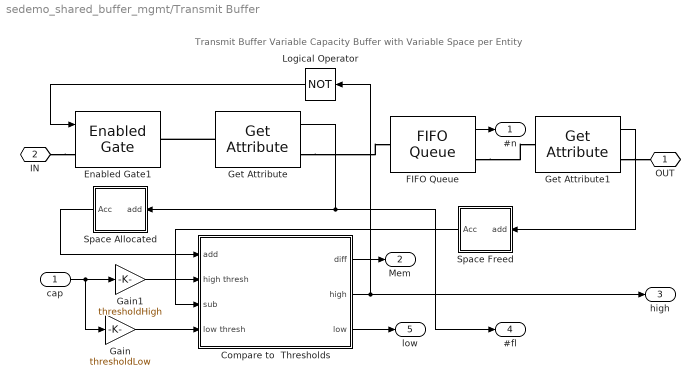
== system sedemo_shared_buffer_mgmt/Transmit Buffer ==
  note: Transmit Buffer
      | Variable Capacity Buffer with Variable Space per Entity
  cap : Inport  OutDataType=sfix(16)  OutScaling=2^0
  Compare to  Thresholds : Subsystem  LoadFcn=des_subsystemblock(gcb, 'load');  InitFcn=des_subsystemblock(gcb, 'init');  StartFcn=des_subsystemblock(gcb, 'start');  StopFcn=des_subsystemblock(gcb, 'stop');
      settings: CopyFcn=des_subsystemblock(gcb, 'copy');  DeleteFcn=des_subsystemblock(gcb, 'delete');  UndoDeleteFcn=des_subsystemblock(gcb, 'undodelete');  ModelCloseFcn=des_subsystemblock(gcb, 'modelclose');  PreSaveFcn=des_subsystemblock(gcb, 'presave');  NameChangeFcn=des_subsystemblock(gcb, 'namechange');  ParentCloseFcn=des_subsystemblock(gcb, 'parentclose');  ErrorFcn=des_subsystemerror
  Enabled Gate1 : simeventsgates1/Enabled Gate  Priority=1  SystemSampleTime=-1  SpecifyEventPriority=off  PriorityGateEnableOpenClose=500  StatNumberDeparted=Off
  FIFO Queue : simeventsqueue1/FIFO Queue  Priority=1  SystemSampleTime=-1  Capacity=inf  EnableTOPort=off  StatNumberDeparted=Off  StatNumberInBlock=On  StatPendingEntity=Off  StatAverageWait=Off  StatAverageQueueLength=Off  StatNumberTimedout=Off
  Gain : Gain  Gain=thresholdLow  ParameterDataType=sfix(16)  ParameterScaling=2^0  OutDataType=sfix(16)  OutScaling=2^0
  Gain1 : Gain  Gain=thresholdHigh  ParameterDataType=sfix(16)  ParameterScaling=2^0  OutDataType=sfix(16)  OutScaling=2^0
  Get Attribute : simeventsattributes2/Get Attribute  Priority=1  DialogController=des_ddg_create  DialogControllerArgs=DataTag125  SystemSampleTime=-1  AttributeName=space  AttributeMissing=Error  AttributeDefaultValue=1  AttributeSendTiming=After entity departure  AttributeTreatAsVector=1  StatNumberDeparted=Off  EvaluatedDefaultAttributeValue={[]}
  Get Attribute1 : simeventsattributes2/Get Attribute  Priority=1  DialogController=des_ddg_create  DialogControllerArgs=DataTag127  SystemSampleTime=-1  AttributeName=space  AttributeMissing=Error  AttributeDefaultValue=1  AttributeSendTiming=After entity departure  AttributeTreatAsVector=1  StatNumberDeparted=Off  EvaluatedDefaultAttributeValue={[]}
  Logical Operator : Logic  Operator=NOT  AllPortsSameDT=off  OutDataTypeMode=Specify via dialog  LogicDataType=float('double')  OutDataTypeStr=float('double')
  Space Allocated : Subsystem  LoadFcn=des_subsystemblock(gcb, 'load');  InitFcn=des_subsystemblock(gcb, 'init');  StartFcn=des_subsystemblock(gcb, 'start');  StopFcn=des_subsystemblock(gcb, 'stop');
      settings: CopyFcn=des_subsystemblock(gcb, 'copy');  DeleteFcn=des_subsystemblock(gcb, 'delete');  UndoDeleteFcn=des_subsystemblock(gcb, 'undodelete');  ModelCloseFcn=des_subsystemblock(gcb, 'modelclose');  PreSaveFcn=des_subsystemblock(gcb, 'presave');  NameChangeFcn=des_subsystemblock(gcb, 'namechange');  ParentCloseFcn=des_subsystemblock(gcb, 'parentclose');  ErrorFcn=des_subsystemerror
  Space Freed : Subsystem  LoadFcn=des_subsystemblock(gcb, 'load');  InitFcn=des_subsystemblock(gcb, 'init');  StartFcn=des_subsystemblock(gcb, 'start');  StopFcn=des_subsystemblock(gcb, 'stop');
      settings: CopyFcn=des_subsystemblock(gcb, 'copy');  DeleteFcn=des_subsystemblock(gcb, 'delete');  UndoDeleteFcn=des_subsystemblock(gcb, 'undodelete');  ModelCloseFcn=des_subsystemblock(gcb, 'modelclose');  PreSaveFcn=des_subsystemblock(gcb, 'presave');  NameChangeFcn=des_subsystemblock(gcb, 'namechange');  ParentCloseFcn=des_subsystemblock(gcb, 'parentclose');  ErrorFcn=des_subsystemerror
  OUT : PMIOPort  Port=1  Side=Right
  IN : PMIOPort  Port=2  Side=Left
  #n : Outport  OutDataType=sfix(16)  OutScaling=2^0
  Mem : Outport  Port=2  OutDataType=sfix(16)  OutScaling=2^0
  high : Outport  Port=3  OutDataType=sfix(16)  OutScaling=2^0
  #fl : Outport  Port=4  OutDataType=sfix(16)  OutScaling=2^0
  low : Outport  Port=5  OutDataType=sfix(16)  OutScaling=2^0
  wires:
  Get Attribute1/1 -> Space Freed/1(add)
  Get Attribute/1 -> Space Allocated/1(add), #fl/1
  Space Freed/1(Acc) -> Compare to  Thresholds/3(sub)
  Space Allocated/1(Acc) -> Compare to  Thresholds/1(add)
  Compare to  Thresholds/2(high) -> Logical Operator/1, high/1
  FIFO Queue/1 -> #n/1
  Compare to  Thresholds/1(diff) -> Mem/1
  Gain/1 -> Compare to  Thresholds/4(low thresh)
  Compare to  Thresholds/3(low) -> low/1
  cap/1 -> Gain/1, Gain1/1
  Logical Operator/1 -> Enabled Gate1/1
  Gain1/1 -> Compare to  Thresholds/2(high thresh)
  connections:
  Get Attribute/RConn1 -- FIFO Queue/LConn1
  FIFO Queue/RConn1 -- Get Attribute1/LConn1
  Get Attribute1/RConn1 -- OUT/RConn1
  Get Attribute/LConn1 -- Enabled Gate1/RConn1
  IN/RConn1 -- Enabled Gate1/LConn1
